simulink library "Motor"  (R2023a)
settings: Solver=VariableStepAuto  StartTime=0.0  StopTime=10.0  RelTol=1e-3
libraries: autolibpmsminterior x1, autolibpmsmexterior x1
settings Model: Creator=25313  LastModifiedBy=25313

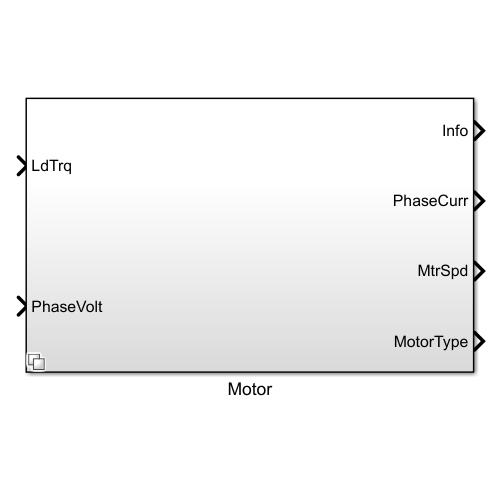
[thumbnail: Simulink's stored preview of the top-level diagram]
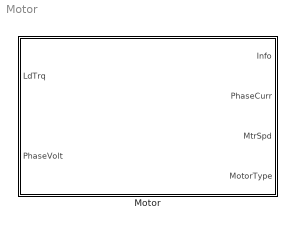
== system Motor ==
  Motor : Subsystem  Variant=on  VariantControl=Choice

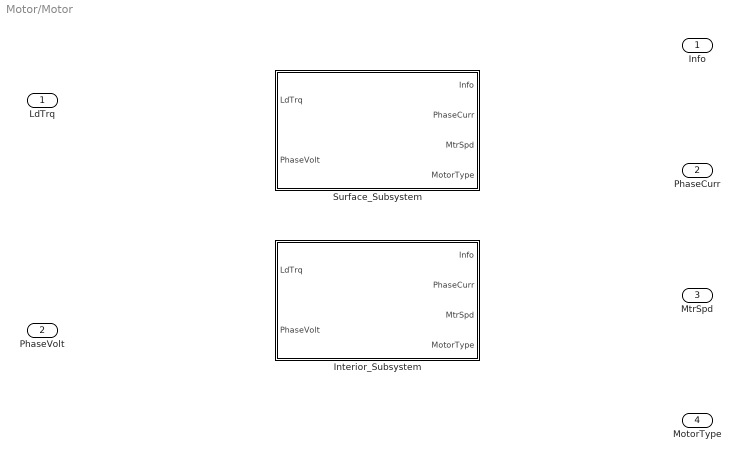
== system Motor/Motor ==
  LdTrq : Inport
  PhaseVolt : Inport  Port=2
  Interior_Subsystem : Subsystem  VariantControl=MotorType == 0
  Surface_Subsystem : Subsystem  VariantControl=MotorType == 1
  Info : Outport
  PhaseCurr : Outport  Port=2
  MtrSpd : Outport  Port=3
  MotorType : Outport  Port=4

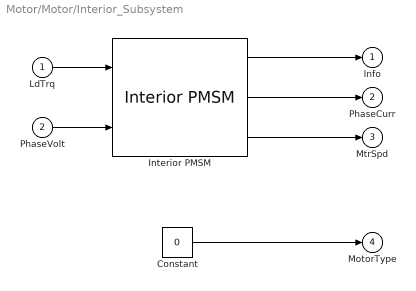
== system Motor/Motor/Interior_Subsystem ==
  LdTrq : Inport
  PhaseVolt : Inport  Port=2
  Constant : Constant  Value=0  OutDataTypeStr=uint8
  Interior PMSM : autolibpmsminterior/Interior PMSM  port_config=Torque  sim_type=Continuous  Ts=0.001  P=4  Rs=0.02  Ldq=[1.7e-3 3.2e-3]  KConstText=Permanent flux linkage constant (lambda_pm):  lambda_pm=0.2205  Ke=159.9771  mechanical=[0.002700,4.924e-4,0]  idq0=[0 0]  theta_init=0  omega_init=0  KConst=0.2205  lambda_pm_calc=0.2205  Kt=0.07  RefBlkName='autolibpmsminterior/Interior PMSM'  aMode=5
      settings: LibrarySourceBlock=mcblib/Electrical Systems/Motors/Interior PMSM
  Info : Outport
  PhaseCurr : Outport  Port=2
  MtrSpd : Outport  Port=3
  MotorType : Outport  Port=4
  wires:
  LdTrq/1 -> Interior PMSM/1
  PhaseVolt/1 -> Interior PMSM/2
  Interior PMSM/1 -> Info/1
  Interior PMSM/2 -> PhaseCurr/1
  Interior PMSM/3 -> MtrSpd/1
  Constant/1 -> MotorType/1

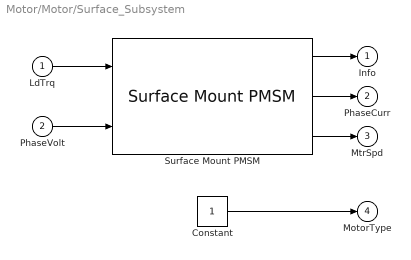
== system Motor/Motor/Surface_Subsystem ==
  LdTrq : Inport
  PhaseVolt : Inport  Port=2
  Constant : Constant  OutDataTypeStr=uint8
  Surface Mount PMSM : autolibpmsmexterior/Surface Mount PMSM  port_config=Torque  sim_type=Continuous  Ts=0.001  P=4  Rs=0.02  Ldq_=1.7e-3  KConstText=Permanent flux linkage constant (lambda_pm):  lambda_pm=0.2205  Ke=159.9771  Kt=1.323  mechanical=[0.0027, 4.924e-4, 0]  idq0=[0 0]  theta_init=0  omega_init=0  KConst=0.2205  lambda_pm_calc=0.2205  RefBlkName='autolibpmsmexterior/Surface Mount PMSM'  aMode=5  Ldq="[0.0017      0.0017]"
  Info : Outport
  PhaseCurr : Outport  Port=2
  MtrSpd : Outport  Port=3
  MotorType : Outport  Port=4
  wires:
  Surface Mount PMSM/1 -> Info/1
  Surface Mount PMSM/2 -> PhaseCurr/1
  Surface Mount PMSM/3 -> MtrSpd/1
  LdTrq/1 -> Surface Mount PMSM/1
  PhaseVolt/1 -> Surface Mount PMSM/2
  Constant/1 -> MotorType/1
